simulink model "L07"  (R2020b)
settings: Solver=FixedStepDiscrete  StartTime=0.0  StopTime=40.0  FixedStep=1  RelTol=1e-3
undefined symbols (not defined in the file): a, b
settings Model: Creator=Nic  LastModifiedBy=Nic

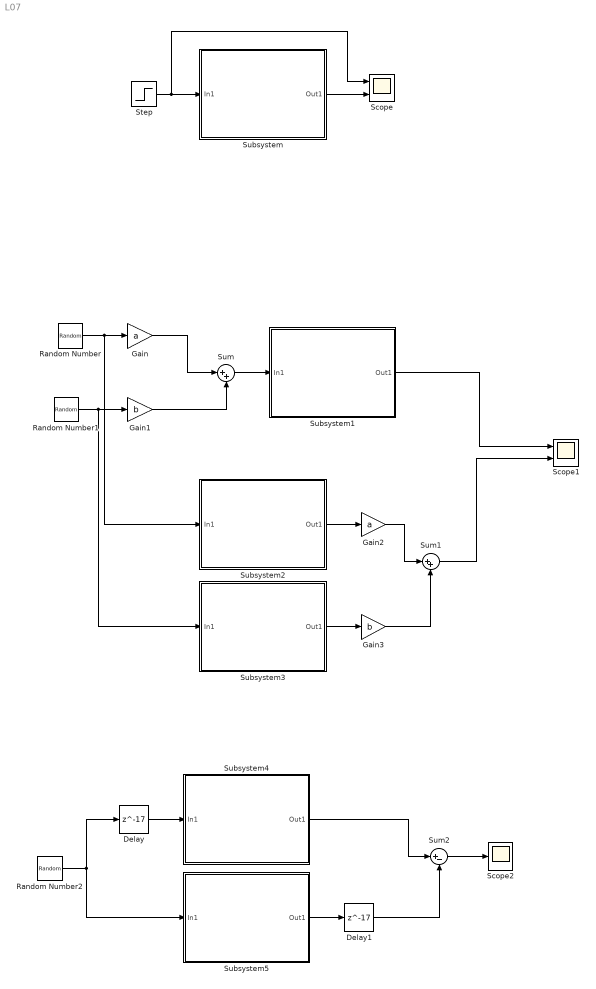
== system L07 ==
  Delay : Delay  DelayLength=17  InitialCondition=0
  Delay1 : Delay  DelayLength=17  InitialCondition=0
  Gain : Gain  Gain=a
  Gain1 : Gain  Gain=b
  Gain2 : Gain  Gain=a
  Gain3 : Gain  Gain=b
  Random Number : RandomNumber  SampleTime=1
  Random Number1 : RandomNumber  Seed=76534  SampleTime=1
  Random Number2 : RandomNumber  SampleTime=1
  Scope : Scope  NumInputPorts=2
  Scope1 : Scope  NumInputPorts=2
  Scope2 : Scope
  Step : Step  SampleTime=0
  Subsystem : Subsystem
  Subsystem1 : Subsystem
  Subsystem2 : Subsystem
  Subsystem3 : Subsystem
  Subsystem4 : Subsystem
  Subsystem5 : Subsystem
  Sum : Sum  Inputs=|++
  Sum1 : Sum  Inputs=|++
  Sum2 : Sum  Inputs=|+-
  wires:
  Step/1 -> Scope/1, Subsystem/1(In1)
  Subsystem/1(Out1) -> Scope/2
  Random Number/1 -> Subsystem2/1(In1), Gain/1
  Random Number1/1 -> Subsystem3/1(In1), Gain1/1
  Gain/1 -> Sum/1
  Gain1/1 -> Sum/2
  Sum/1 -> Subsystem1/1(In1)
  Subsystem1/1(Out1) -> Scope1/1
  Subsystem2/1(Out1) -> Gain2/1
  Subsystem3/1(Out1) -> Gain3/1
  Gain2/1 -> Sum1/1
  Gain3/1 -> Sum1/2
  Sum1/1 -> Scope1/2
  Delay/1 -> Subsystem4/1(In1)
  Subsystem4/1(Out1) -> Sum2/1
  Random Number2/1 -> Delay/1, Subsystem5/1(In1)
  Subsystem5/1(Out1) -> Delay1/1
  Delay1/1 -> Sum2/2
  Sum2/1 -> Scope2/1

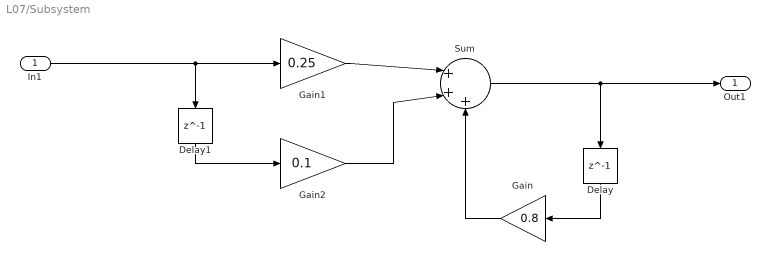
== system L07/Subsystem ==
  In1 : Inport
  Delay : Delay  DelayLength=1  InitialCondition=0
  Delay1 : Delay  DelayLength=1  InitialCondition=0
  Gain : Gain  Gain=0.8
  Gain1 : Gain  Gain=0.25
  Gain2 : Gain  Gain=0.1
  Sum : Sum  Inputs=|+++
  Out1 : Outport
  wires:
  Delay/1 -> Gain/1
  In1/1 -> Delay1/1, Gain1/1
  Sum/1 -> Out1/1, Delay/1
  Gain/1 -> Sum/3
  Gain2/1 -> Sum/2
  Delay1/1 -> Gain2/1
  Gain1/1 -> Sum/1

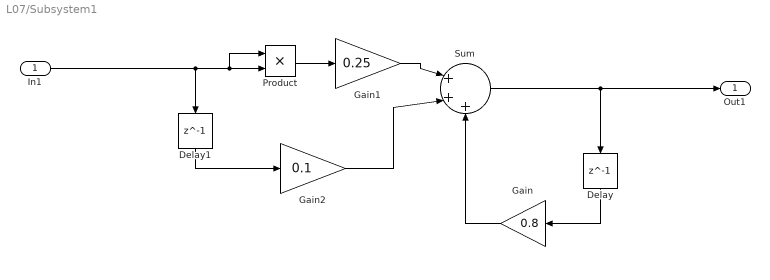
== system L07/Subsystem1 ==
  In1 : Inport
  Delay : Delay  DelayLength=1  InitialCondition=0
  Delay1 : Delay  DelayLength=1  InitialCondition=0
  Gain : Gain  Gain=0.8
  Gain1 : Gain  Gain=0.25
  Gain2 : Gain  Gain=0.1
  Product : Product
  Sum : Sum  Inputs=|+++
  Out1 : Outport
  wires:
  Delay/1 -> Gain/1
  In1/1 -> Delay1/1, Product/1, Product/2
  Sum/1 -> Out1/1, Delay/1
  Gain/1 -> Sum/3
  Gain2/1 -> Sum/2
  Delay1/1 -> Gain2/1
  Gain1/1 -> Sum/1
  Product/1 -> Gain1/1

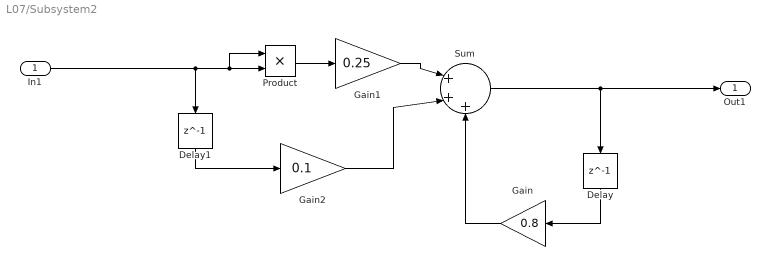
== system L07/Subsystem2 ==
  In1 : Inport
  Delay : Delay  DelayLength=1  InitialCondition=0
  Delay1 : Delay  DelayLength=1  InitialCondition=0
  Gain : Gain  Gain=0.8
  Gain1 : Gain  Gain=0.25
  Gain2 : Gain  Gain=0.1
  Product : Product
  Sum : Sum  Inputs=|+++
  Out1 : Outport
  wires:
  Delay/1 -> Gain/1
  In1/1 -> Delay1/1, Product/1, Product/2
  Sum/1 -> Out1/1, Delay/1
  Gain/1 -> Sum/3
  Gain2/1 -> Sum/2
  Delay1/1 -> Gain2/1
  Gain1/1 -> Sum/1
  Product/1 -> Gain1/1

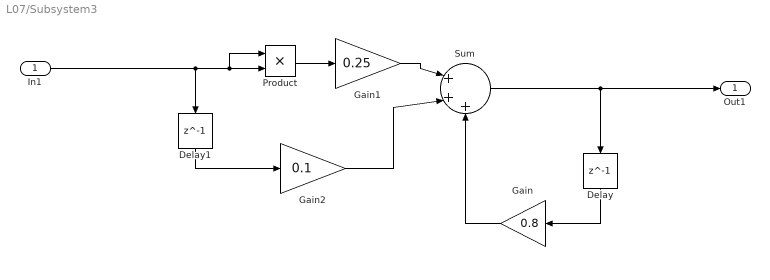
== system L07/Subsystem3 ==
  In1 : Inport
  Delay : Delay  DelayLength=1  InitialCondition=0
  Delay1 : Delay  DelayLength=1  InitialCondition=0
  Gain : Gain  Gain=0.8
  Gain1 : Gain  Gain=0.25
  Gain2 : Gain  Gain=0.1
  Product : Product
  Sum : Sum  Inputs=|+++
  Out1 : Outport
  wires:
  Delay/1 -> Gain/1
  In1/1 -> Delay1/1, Product/1, Product/2
  Sum/1 -> Out1/1, Delay/1
  Gain/1 -> Sum/3
  Gain2/1 -> Sum/2
  Delay1/1 -> Gain2/1
  Gain1/1 -> Sum/1
  Product/1 -> Gain1/1

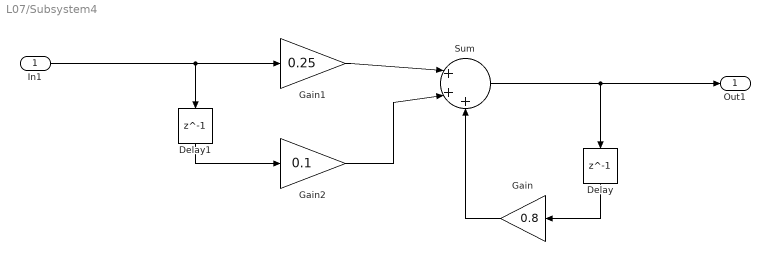
== system L07/Subsystem4 ==
  In1 : Inport
  Delay : Delay  DelayLength=1  InitialCondition=0
  Delay1 : Delay  DelayLength=1  InitialCondition=0
  Gain : Gain  Gain=0.8
  Gain1 : Gain  Gain=0.25
  Gain2 : Gain  Gain=0.1
  Sum : Sum  Inputs=|+++
  Out1 : Outport
  wires:
  Delay/1 -> Gain/1
  In1/1 -> Delay1/1, Gain1/1
  Sum/1 -> Out1/1, Delay/1
  Gain/1 -> Sum/3
  Gain2/1 -> Sum/2
  Delay1/1 -> Gain2/1
  Gain1/1 -> Sum/1

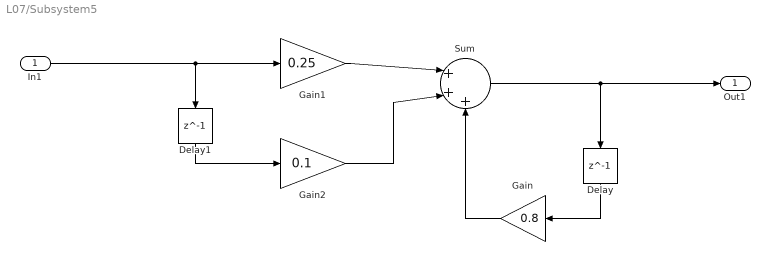
== system L07/Subsystem5 ==
  In1 : Inport
  Delay : Delay  DelayLength=1  InitialCondition=0
  Delay1 : Delay  DelayLength=1  InitialCondition=0
  Gain : Gain  Gain=0.8
  Gain1 : Gain  Gain=0.25
  Gain2 : Gain  Gain=0.1
  Sum : Sum  Inputs=|+++
  Out1 : Outport
  wires:
  Delay/1 -> Gain/1
  In1/1 -> Delay1/1, Gain1/1
  Sum/1 -> Out1/1, Delay/1
  Gain/1 -> Sum/3
  Gain2/1 -> Sum/2
  Delay1/1 -> Gain2/1
  Gain1/1 -> Sum/1
